simulink model "computeF"  (Simulink 7.9)
settings: Solver=FixedStepDiscrete  StartTime=0.0  StopTime=1000  FixedStep=0.01  RelTol=1e-3
PreLoadFcn:
  | robotName = 'icubGazeboSim';
  | localName = 'SimulinkiCubGazeboSim';
InitFcn:
  | robotName = 'icubGazeboSim';
  | localName = 'SimulinkiCubGazeboSim';
libraries: WBCLibrary x14
settings Model: Creator=iron  LastModifiedBy=jorhabib
settings DebuggingCC: FcnCallInpInsideContextMsg=Use local settings
settings CodeAppCC: CustomSymbolStrType=$N$R$M_T
settings GRTTargetCC: CodeReplacementLibrary=C89/C90 (ANSI)  CombineOutputUpdateFcns=off  GRTInterface=on

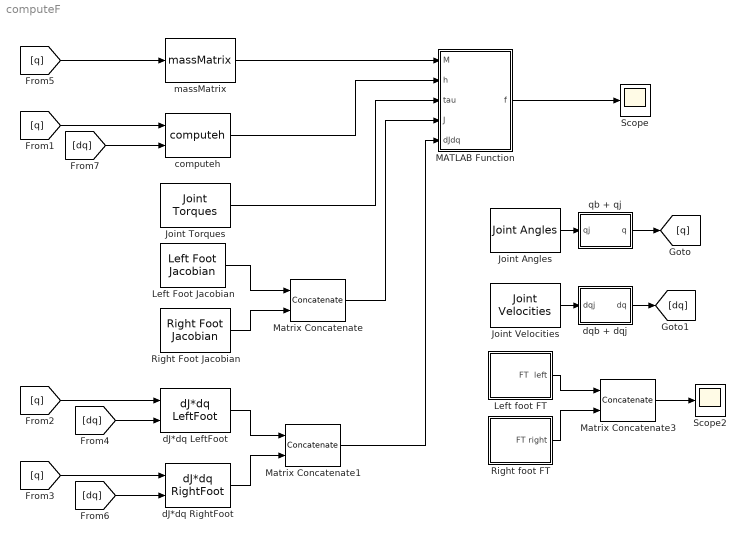
== system computeF ==
  Joint Angles : WBCLibrary/wholeBodyStates/Joint Angles  robotName=robotName  localName=localName
  Joint Torques : WBCLibrary/wholeBodyStates/Joint Torques  robotName=robotName  localName=localName
  Joint Velocities : WBCLibrary/wholeBodyStates/Joint Velocities  robotName=robotName  localName=localName
  Left Foot Jacobian : WBCLibrary/wholeBodyModel/Jacobians/Left Foot Jacobian  robotName=robotName  localName=localName
  Left foot FT : Subsystem
  MATLAB Function : MATLAB Function  TreatAsAtomicUnit=on
      settings: PermitHierarchicalResolution=ParametersOnly
  Matrix Concatenate : Concatenate  Mode=Multidimensional array
  Matrix Concatenate1 : Concatenate  Mode=Multidimensional array
  Matrix Concatenate3 : Concatenate  Mode=Multidimensional array
  Right Foot Jacobian : WBCLibrary/wholeBodyModel/Jacobians/Right Foot Jacobian  robotName=robotName  localName=localName
  Right foot FT : Subsystem
  Scope : Scope
      settings: TimeRange=0.9  YMin=-20  YMax=160
  Scope2 : Scope
      settings: TimeRange=0.9  YMin=-10  YMax=120
  computeh : WBCLibrary/wholeBodyModel/Dynamics/computeh  val=7  robotname=robotName  localname=localName
  dJ*dq LeftFoot : WBCLibrary/wholeBodyModel/Dynamics/dJ*dq LeftFoot  val=9  robotName=robotName  localName=localName
  dJ*dq RightFoot : WBCLibrary/wholeBodyModel/Dynamics/dJ*dq RightFoot  val=9  robotName=robotName  localName=localName
  dqb + dqj : Subsystem
  massMatrix : WBCLibrary/wholeBodyModel/Dynamics/massMatrix  val=8  robotname=robotName  localname=localName
  qb + qj : Subsystem
  wires:
  massMatrix/1 -> MATLAB Function/1(M)
  computeh/1 -> MATLAB Function/2(h)
  Left Foot Jacobian/1 -> Matrix Concatenate/1
  Right Foot Jacobian/1 -> Matrix Concatenate/2
  Matrix Concatenate/1 -> MATLAB Function/4(J)
  dJ*dq LeftFoot/1 -> Matrix Concatenate1/1
  dJ*dq RightFoot/1 -> Matrix Concatenate1/2
  Matrix Concatenate1/1 -> MATLAB Function/5(dJdq)
  MATLAB Function/1(f) -> Scope/1
  Left foot FT/1(FT  left) -> Matrix Concatenate3/1
  Right foot FT/1(FT right) -> Matrix Concatenate3/2
  Matrix Concatenate3/1 -> Scope2/1
  Joint Angles/1 -> qb + qj/1(qj)
  Joint Velocities/1 -> dqb + dqj/1(dqj)
  qb + qj/1(q) -> [q]
  dqb + dqj/1(dq) -> [dq]
  [q] -> massMatrix/1
  [q] -> computeh/1
  [q] -> dJ*dq LeftFoot/1
  [q] -> dJ*dq RightFoot/1
  [dq] -> computeh/2
  [dq] -> dJ*dq LeftFoot/2
  [dq] -> dJ*dq RightFoot/2
  Joint Torques/1 -> MATLAB Function/3(tau)

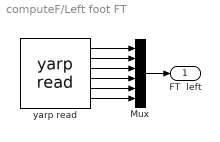
== system computeF/Left foot FT ==
  Mux : Mux  Inputs=6
  yarp read : WBCLibrary/Utilities/yarp read  from=['/' robotName '/left_foot/analog:o']  to='/left_foot/FT'  num=6  blocking=off  timestamp=off
  FT  left : Outport
  wires:
  yarp read/1 -> Mux/1
  yarp read/2 -> Mux/2
  yarp read/3 -> Mux/3
  yarp read/4 -> Mux/4
  yarp read/5 -> Mux/5
  yarp read/6 -> Mux/6
  Mux/1 -> FT  left/1

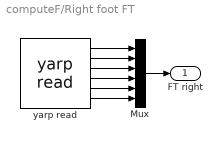
== system computeF/Right foot FT ==
  Mux : Mux  Inputs=6
  yarp read : WBCLibrary/Utilities/yarp read  from=['/' robotName '/right_foot/analog:o']  to='/right_foot/FT'  num=6  blocking=off  timestamp=off
  FT right : Outport
  wires:
  yarp read/1 -> Mux/1
  yarp read/2 -> Mux/2
  yarp read/3 -> Mux/3
  yarp read/4 -> Mux/4
  yarp read/5 -> Mux/5
  yarp read/6 -> Mux/6
  Mux/1 -> FT right/1

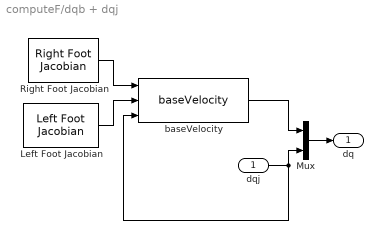
== system computeF/dqb + dqj ==
  dqj : Inport
  Left Foot Jacobian : WBCLibrary/wholeBodyModel/Jacobians/Left Foot Jacobian  robotName=robotName  localName=localName
  Mux : Mux  Inputs=2
  Right Foot Jacobian : WBCLibrary/wholeBodyModel/Jacobians/Right Foot Jacobian  robotName=robotName  localName=localName
  baseVelocity : WBCLibrary/Utilities/baseVelocity
  dq : Outport
  wires:
  Left Foot Jacobian/1 -> baseVelocity/2
  Right Foot Jacobian/1 -> baseVelocity/1
  baseVelocity/1 -> Mux/1
  dqj/1 -> baseVelocity/3, Mux/2
  Mux/1 -> dq/1

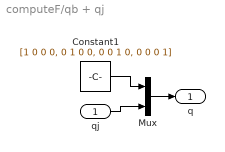
== system computeF/qb + qj ==
  qj : Inport
  Constant1 : Constant  Value=[1 0 0 0, 0 1 0 0, 0 0 1 0, 0 0 0 1]
  Mux : Mux  Inputs=2
  q : Outport
  wires:
  Mux/1 -> q/1
  qj/1 -> Mux/2
  Constant1/1 -> Mux/1

== matlab function MATLAB Function ==
  data: M input double; f output double; h input double; tau input double; J input double; dJdq input double
function f  = fcn(M, h, tau, J, dJdq)

% Francesco Nori
% Genova 6 Marzo 2014
% CODYCO project
%
% This code computes the forces f acting on a kinematic chain
% subject to a set of constraints. The kinematic chain dynamics
% are described as follows:
%
% M d2q + h - J' f = tau  
%
% The constraints are described in a differential form:
%
% J dq = 0
%
% whose derivative is:
%
% dJ dq  + J d2q = 0
%

S = [zeros(25,6) eye(25)];
Minv = inv(M);
f = -(J*Minv*J')\(J*Minv*(S'*tau - h)+ dJdq);
